simulink model "req19C"  (R2019a)
settings: Solver=FixedStepAuto  StartTime=0.0  StopTime=100  RelTol=1e-3
libraries: simulink x8
settings Model: Creator=e40014285  LastModifiedBy=e40014285
settings ConfigComp: CovScope=ReferencedModels  CovIncludeTopModel=off  CovHTMLOptions=-sRT=1 -sVT=0 -aTS=1 -bRG=1 -bTC=1 -hTR=0 -nFC=0 -nFD=1 -scm=1 -bcm=1 -xEv=0 -xEM=0  CovHtmlReporting=on  CovCumulativeReport=on  DVMaxProcessTime=6000  DVModelCoverageObjectives=EnhancedMCDC  DVTestSuiteOptimization=Auto  DVDetectOutOfBounds=on  DVReportPDFFormat=on  DVRebuildModelRepresentation=Always

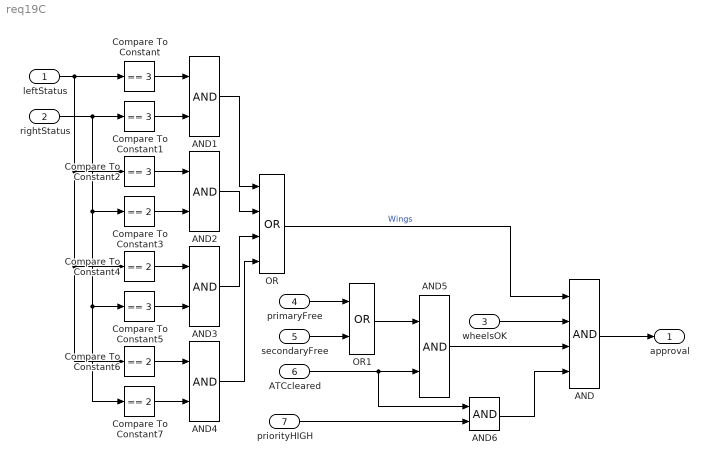
== system req19C ==
  leftStatus : Inport
  rightStatus : Inport  Port=2
  wheelsOK : Inport  Port=3
  primaryFree : Inport  Port=4
  secondaryFree : Inport  Port=5
  ATCcleared : Inport  Port=6
  priorityHIGH : Inport  Port=7
  AND : Logic  Inputs=4  AllPortsSameDT=off  OutDataTypeStr=boolean
  AND{1..6} (6 alike) : Logic  AllPortsSameDT=off  OutDataTypeStr=boolean
  Compare To Constant{,1..2,5} (4 alike) : simulink/Logic and Bit Operations/Compare To Constant  relop===  const=3  OutDataTypeStr=boolean
  Compare To Constant{3..4,6..7} (4 alike) : simulink/Logic and Bit Operations/Compare To Constant  relop===  const=2  OutDataTypeStr=boolean
  OR : Logic  Operator=OR  Inputs=4  AllPortsSameDT=off  OutDataTypeStr=boolean
  OR1 : Logic  Operator=OR  AllPortsSameDT=off  OutDataTypeStr=boolean
  approval : Outport
  wires:
  AND/1 -> approval/1
  OR/1 -> AND/1  "Wings"
  leftStatus/1 -> Compare To Constant2/1, Compare To Constant4/1, Compare To Constant6/1, Compare To Constant/1
  rightStatus/1 -> Compare To Constant7/1, Compare To Constant5/1, Compare To Constant3/1, Compare To Constant1/1
  Compare To Constant/1 -> AND1/1
  Compare To Constant1/1 -> AND1/2
  AND1/1 -> OR/1
  Compare To Constant3/1 -> AND2/2
  Compare To Constant2/1 -> AND2/1
  Compare To Constant4/1 -> AND3/1
  Compare To Constant5/1 -> AND3/2
  AND2/1 -> OR/2
  AND3/1 -> OR/3
  Compare To Constant7/1 -> AND4/2
  Compare To Constant6/1 -> AND4/1
  AND4/1 -> OR/4
  wheelsOK/1 -> AND/2
  primaryFree/1 -> OR1/1
  secondaryFree/1 -> OR1/2
  OR1/1 -> AND5/1
  ATCcleared/1 -> AND6/1, AND5/2
  AND5/1 -> AND/3
  priorityHIGH/1 -> AND6/2
  AND6/1 -> AND/4
